simulink model "sensor_diagnosis"  (R2018b)
settings: Solver=FixedStepAuto  StartTime=0.0  StopTime=2000  FixedStep=0.02  RelTol=1e-3
values from neighbouring files (symbols this model uses):
  R = 0.003*eye(size(C,1))    [Com_of_kalman_gain.m]    (also in Copy_of_kalman_gain.m = diag(y_noise.^2); MM_HKF.m = diag(y_svar.^2); MM_based.m = diag(y_svar.^2); act_fault_of_kalman_gain.m = 0.02^2*eye(size(C,1)))
undefined symbols (not defined in the file or in its folder): piece
libraries: sharedschedule x121, dspsigattribs x22, commchan3 x1, dsparch4 x1, simulink x1
(part 1 of 2)
settings Model: Creator=mmm  LastModifiedBy=ma

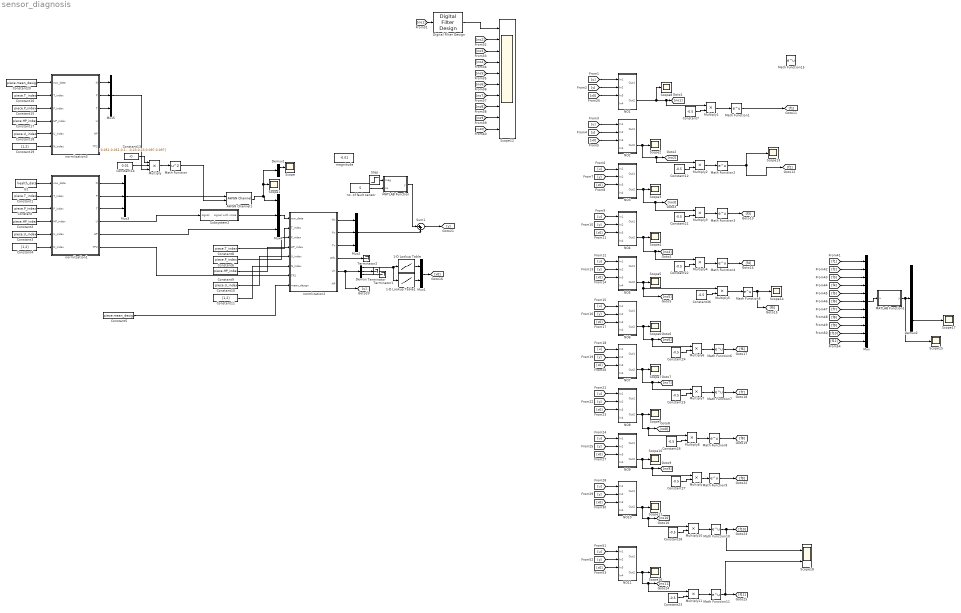
== system sensor_diagnosis ==
  1-D Lookup Table : Lookup_n-D  NumberOfTableDimensions=1  BreakpointsForDimension1=piece.Wf_stable_(:,1)  Table=piece.Nl  InterpMethod=Cubic spline  ExtrapMethod=Cubic spline  InternalRulePriority=Speed  RndMeth=Simplest  InputSameDT=on
  1-D Lookup Table1 : Lookup_n-D  NumberOfTableDimensions=1  BreakpointsForDimension1=piece.Wf_stable_(:,1)  Table=piece.N_stable_(:,2)  InterpMethod=Cubic spline  ExtrapMethod=Cubic spline  InternalRulePriority=Speed  RndMeth=Simplest  InputSameDT=on
  AWGN Channel1 : commchan3/AWGN Channel  InputProcessing=Columns as channels (frame based)  seed=11:20  noiseMode=Variance from port  EbNodB=10  EsNodB=10  SNRdB=10  bitsPerSym=1  Ps=1  Tsym=1  variance=[2.55,7.5,0.03,0.03,0.3,0.3,0.15,0.15,0.45,0.45].^2
  Constant : Constant  Value=piece.P_index  VectorParams1D=off
  Constant1 : Constant  Value=piece.T_index  VectorParams1D=off
  Constant10 : Constant  Value=piece.U_index  VectorParams1D=off
  Constant11 : Constant  Value=[1,2]  VectorParams1D=off
  Constant{7,12,21..28,36} (11 alike) : Constant  Value=-0.5
  Constant13 : Constant  Value=[0.051,0.051,0.164,0.164,0.15,0.15,0.23,0.23,0.097,0.097]
  Constant14 : Constant  Value=0.01
  Constant15 : Constant  Value=piece.P_index  VectorParams1D=off
  Constant16 : Constant  Value=piece.T_index  VectorParams1D=off
  Constant17 : Constant  Value=piece.HP_index  VectorParams1D=off
  Constant18 : Constant  Value=piece.U_index  VectorParams1D=off
  Constant19 : Constant  Value=[1,2]  VectorParams1D=off
  Constant2 : Constant  Value=piece.HP_index  VectorParams1D=off
  Constant20 : Constant  Value=piece.mean_design  VectorParams1D=off
  Constant3 : Constant  Value=piece.U_index  VectorParams1D=off
  Constant4 : Constant  Value=[1,2]  VectorParams1D=off
  Constant5 : Constant  Value=piece.mean_design  VectorParams1D=off
  Constant6 : Constant  Value=piece.P_index  VectorParams1D=off
  Constant8 : Constant  Value=piece.T_index  VectorParams1D=off
  Constant9 : Constant  Value=piece.HP_index  VectorParams1D=off
  Demux : Demux  Outputs=3
  Demux1 : Demux  Outputs=[1,9]
  Demux2 : Demux  Outputs=10
  Digital Filter Design : dsparch4/Digital Filter Design  mwdsp_browser_bugfix_var=off
  MATLAB Function : MATLAB Function  TreatAsAtomicUnit=on
  MATLAB Function1 : MATLAB Function  TreatAsAtomicUnit=on
  Math Function : Math  Operator=square  SaturateOnIntegerOverflow=on
  Math Function{1..11,15} (12 alike) : Math  SaturateOnIntegerOverflow=on
  Multiply : Product  Inputs=3
  Multiply{1..11} (11 alike) : Product
  Mux : Mux  Inputs=11
  Mux1 : Mux  Inputs=2
  Mux{2..5} (4 alike) : Mux  Inputs=3
  NO1 : Subsystem
  NO10 : Subsystem
  NO11 : Subsystem
  NO2 : Subsystem
  NO3 : Subsystem
  NO4 : Subsystem
  NO5 : Subsystem
  NO6 : Subsystem
  NO7 : Subsystem
  NO8 : Subsystem
  NO9 : Subsystem
  Scope{,1..11,13..17} (17 alike) : Scope
  Scope12 : Scope  NumInputPorts=10
  Scope18 : Scope  NumInputPorts=2
  Step : Step  Time=300  After=-0.02  SampleTime=0
  Subsystem2 : Subsystem
  Sum1 : Sum  Inputs=|++
  Terminator : Terminator
  Terminator1 : Terminator
  Terminator2 : Terminator
  U2 : FromWorkspace  VariableName=health_data  SampleTime=0.02  Interpolate=off  OutputAfterFinalValue=Holding final value
  magnitude : Constant  Value=-0.01
  no. of fault sensor : Constant  Value=5
  normlization1 : MATLAB Function  TreatAsAtomicUnit=on
  normlization2 : MATLAB Function  TreatAsAtomicUnit=on
  normlization3 : MATLAB Function  TreatAsAtomicUnit=on
  wires:
  Constant4/1 -> normlization1/6(N_index)
  Constant2/1 -> normlization1/4(HP_index)
  Constant3/1 -> normlization1/5(U_index)
  Constant1/1 -> normlization1/2(T_index)
  U2/1 -> normlization1/1(row_data)
  Constant/1 -> normlization1/3(P_index)
  Demux/1 -> 1-D Lookup Table1/1, 1-D Lookup Table/1
  Demux/2 -> Terminator/1
  Demux/3 -> Terminator1/1
  1-D Lookup Table/1 -> Mux1/1
  1-D Lookup Table1/1 -> Mux1/2
  Mux1/1 -> [x0]
  normlization2/5(Un) -> Demux/1, [u]
  Mux2/1 -> Sum1/2
  Sum1/1 -> [y]
  normlization1/1(N) -> Mux3/1
  normlization1/2(P) -> Mux3/2
  normlization1/3(T) -> Mux3/3
  Constant5/1 -> normlization2/8(mean_design)
  Mux3/1 -> AWGN Channel1/1
  normlization1/5(HP) -> Mux4/3
  Mux4/1 -> normlization2/1(row_data)
  Constant8/1 -> normlization2/2(T_index)
  Constant6/1 -> normlization2/3(P_index)
  Constant9/1 -> normlization2/4(HP_index)
  Constant10/1 -> normlization2/5(U_index)
  Constant11/1 -> normlization2/6(N_index)
  normlization2/1(Nn) -> Mux2/1
  normlization2/2(Pn) -> Mux2/2
  normlization2/3(Tn) -> Mux2/3
  normlization1/4(U) -> Subsystem2/1(signal)
  Subsystem2/1(signal with noise) -> Mux4/2
  normlization2/4(Wfn) -> Terminator2/1
  normlization1/6(TP2) -> normlization2/7(TP2)
  Demux1/1 -> Scope/1
  Constant13/1 -> Multiply/1
  Constant14/1 -> Multiply/2
  Multiply/1 -> Math Function/1
  Math Function/1 -> AWGN Channel1/2
  AWGN Channel1/1 -> Scope1/1, Demux1/1, Mux4/1
  Constant15/1 -> normlization3/3(P_index)
  Constant20/1 -> normlization3/1(row_data)
  Constant16/1 -> normlization3/2(T_index)
  Constant18/1 -> normlization3/5(U_index)
  Constant17/1 -> normlization3/4(HP_index)
  Constant19/1 -> normlization3/6(N_index)
  normlization3/1(N) -> Mux5/1
  normlization3/2(P) -> Mux5/2
  normlization3/3(T) -> Mux5/3
  Mux5/1 -> Multiply/3
  [u] -> NO1/1(In1)
  [y] -> NO1/2(In2)
  [x0] -> NO1/3(In3)
  NO1/2(Out2) -> Scope8/1, Multiply1/1, [no1]
  [u] -> NO2/1(In1)
  [y] -> NO2/2(In2)
  [x0] -> NO2/3(In3)
  [u] -> NO3/1(In1)
  [y] -> NO3/2(In2)
  [x0] -> NO3/3(In3)
  [x0] -> NO4/3(In3)
  [y] -> NO4/2(In2)
  [u] -> NO4/1(In1)
  [x0] -> NO5/3(In3)
  [y] -> NO5/2(In2)
  [u] -> NO5/1(In1)
  [x0] -> NO6/3(In3)
  [y] -> NO6/2(In2)
  [u] -> NO6/1(In1)
  [x0] -> NO7/3(In3)
  [y] -> NO7/2(In2)
  [u] -> NO7/1(In1)
  [x0] -> NO8/3(In3)
  [y] -> NO8/2(In2)
  [u] -> NO8/1(In1)
  [x0] -> NO9/3(In3)
  [y] -> NO9/2(In2)
  [u] -> NO9/1(In1)
  [x0] -> NO10/3(In3)
  [y] -> NO10/2(In2)
  [u] -> NO10/1(In1)
  [no2] -> Scope12/2
  [no3] -> Scope12/3
  [no4] -> Scope12/4
  [no5] -> Scope12/5
  [no6] -> Scope12/6
  [no7] -> Scope12/7
  [no8] -> Scope12/8
  [no9] -> Scope12/9
  [no10] -> Scope12/10
  no. of fault sensor/1 -> MATLAB Function/2(no)
  MATLAB Function/1(y) -> Sum1/1
  Step/1 -> MATLAB Function/1(mag)
  Constant7/1 -> Multiply1/2
  Multiply1/1 -> Math Function1/1
  Multiply2/1 -> Math Function2/1
  NO2/2(Out2) -> Multiply2/1, [no2], Scope2/1
  Constant12/1 -> Multiply2/2
  Multiply3/1 -> Math Function3/1
  NO3/2(Out2) -> Multiply3/1, [no3], Scope3/1
  Constant21/1 -> Multiply3/2
  Multiply4/1 -> Math Function4/1
  NO4/2(Out2) -> Multiply4/1, [no4], Scope4/1
  Constant22/1 -> Multiply4/2
  NO5/2(Out2) -> [no5], Multiply5/1, Scope5/1
  Multiply6/1 -> Math Function6/1
  NO6/2(Out2) -> Multiply6/1, [no6], Scope6/1
  Constant24/1 -> Multiply6/2
  Multiply7/1 -> Math Function7/1
  NO7/2(Out2) -> Multiply7/1, [no7], Scope7/1
  Constant25/1 -> Multiply7/2
  Multiply8/1 -> Math Function8/1
  NO8/2(Out2) -> Multiply8/1, [no8], Scope9/1
  Constant26/1 -> Multiply8/2
  Multiply9/1 -> Math Function9/1
  NO9/2(Out2) -> Multiply9/1, [no9], Scope10/1
  Constant27/1 -> Multiply9/2
  Multiply10/1 -> Math Function10/1
  NO10/2(Out2) -> Multiply10/1, [no10], Scope11/1
  Constant28/1 -> Multiply10/2
  Multiply5/1 -> Math Function5/1
  Constant36/1 -> Multiply5/2
  [no1] -> Digital Filter Design/1
  Digital Filter Design/1 -> Scope12/1
  Math Function1/1 -> [f1]
  Math Function5/1 -> [f5], Scope14/1
  Math Function2/1 -> [f2], Scope13/1
  Math Function3/1 -> [f3]
  Math Function4/1 -> [f4]
  Math Function6/1 -> [f6]
  Math Function7/1 -> [f7]
  Math Function8/1 -> [f8]
  Math Function9/1 -> [f9]
  Math Function10/1 -> Scope18/1, [f10]
  [f1] -> Mux/1
  [f2] -> Mux/2
  [f3] -> Mux/3
  [f4] -> Mux/4
  [f5] -> Mux/5
  [f6] -> Mux/6
  [f7] -> Mux/7
  [f8] -> Mux/8
  [f9] -> Mux/9
  [f10] -> Mux/10
  Mux/1 -> MATLAB Function1/1(u)
  MATLAB Function1/1(y) -> Scope15/1, Demux2/1
  Math Function11/1 -> Scope18/2, [f11]
  Constant23/1 -> Multiply11/2
  NO11/2(Out2) -> Scope16/1, [no11], Multiply11/1
  Multiply11/1 -> Math Function11/1
  [y] -> NO11/2(In2)
  [x0] -> NO11/3(In3)
  [u] -> NO11/1(In1)
  [f11] -> Mux/11
  Demux2/9 -> Scope17/1

== system sensor_diagnosis/NO1 ==
  In1 : Inport
  In2 : Inport  Port=2
  In3 : Inport  Port=3
  In4 : Inport  Port=4
  A : sharedschedule/Interpolate Matrix(x)   matrix=piece.A  aMode=aMode
      settings: SourceProductName=Aerospace Blockset  SourceProductBaseCode=AE
  B : sharedschedule/Interpolate Matrix(x)   matrix=piece.B  aMode=aMode
      settings: SourceProductName=Aerospace Blockset  SourceProductBaseCode=AE
  C : sharedschedule/Interpolate Matrix(x)   matrix=piece.C  aMode=aMode
      settings: SourceProductName=Aerospace Blockset  SourceProductBaseCode=AE
  D : sharedschedule/Interpolate Matrix(x)   matrix=piece.D  aMode=aMode
      settings: SourceProductName=Aerospace Blockset  SourceProductBaseCode=AE
  K1 : sharedschedule/Interpolate Matrix(x)   matrix=piece.K_s  aMode=aMode
      settings: SourceProductName=Aerospace Blockset  SourceProductBaseCode=AE
  K2 : sharedschedule/Interpolate Matrix(x)   matrix=piece.S_s  aMode=aMode
      settings: SourceProductName=Aerospace Blockset  SourceProductBaseCode=AE
  L : sharedschedule/Interpolate Matrix(x)   matrix=piece.L  aMode=aMode
      settings: SourceProductName=Aerospace Blockset  SourceProductBaseCode=AE
  M : sharedschedule/Interpolate Matrix(x)   matrix=piece.M  aMode=aMode
      settings: SourceProductName=Aerospace Blockset  SourceProductBaseCode=AE
  Matrix Divide1 : Product  Inputs=*/  Multiplication=Matrix(*)
  MatrixMultiply1 : Product  Multiplication=Matrix(*)
  Minus1 : Sum  Inputs=+-
  Minus5 : Sum  Inputs=+-
  Prelookup : PreLookup  BreakpointsData=piece.Nl  BreakpointObject=Nl  ExtrapMethod=Linear  UseLastBreakpoint=on  DiagnosticForOutOfRangeInput=Warning
  Scope2 : Scope
  Selector : Selector  InputPortWidth=2  IndexOptions=Index vector (dialog)  Indices=[1]  OutputSizes=1
  Transpose3 : Math  Operator=transpose  SaturateOnIntegerOverflow=on
  kalman filter1 : Subsystem
  steadyOutput : sharedschedule/Interpolate Matrix(x)   matrix=piece.steadyOutput  aMode=aMode
      settings: SourceProductName=Aerospace Blockset  SourceProductBaseCode=AE
  steadyState : sharedschedule/Interpolate Matrix(x)   matrix=piece.steadyState  aMode=aMode
      settings: SourceProductName=Aerospace Blockset  SourceProductBaseCode=AE
  steadyinput : sharedschedule/Interpolate Matrix(x)   matrix=piece.steadyInput  aMode=aMode
      settings: SourceProductName=Aerospace Blockset  SourceProductBaseCode=AE
  Out1 : Outport
  Out2 : Outport  Port=2
  wires:
  D/1 -> kalman filter1/4(D)
  Prelookup/1 -> K2/1, K1/1, M/1, L/1, steadyState/1, steadyinput/1, steadyOutput/1, D/1, C/1, B/1, A/1
  In4/1 -> kalman filter1/12(P)
  kalman filter1/3(Y_error) -> Transpose3/1, MatrixMultiply1/2, Scope2/1
  B/1 -> kalman filter1/2(B)
  Prelookup/2 -> A/2, steadyState/2, K2/2, K1/2, M/2, L/2, steadyinput/2, steadyOutput/2, D/2, C/2, B/2
  Selector/1 -> Prelookup/1
  steadyState/1 -> kalman filter1/9(Xtrim)
  Transpose3/1 -> Matrix Divide1/1
  Matrix Divide1/1 -> MatrixMultiply1/1
  L/1 -> kalman filter1/10(L)
  C/1 -> kalman filter1/3(C)
  Minus5/1 -> kalman filter1/7(Y)
  kalman filter1/2(Y_es) -> Out1/1
  Minus1/1 -> kalman filter1/8(U)
  kalman filter1/1(X_es) -> Selector/1
  steadyinput/1 -> Minus1/2
  K1/1 -> kalman filter1/5(K)
  steadyOutput/1 -> Minus5/2
  A/1 -> kalman filter1/1(A)
  MatrixMultiply1/1 -> Out2/1
  M/1 -> kalman filter1/11(M)
  In3/1 -> kalman filter1/6(x0)
  In2/1 -> Minus5/1
  In1/1 -> Minus1/1
  K2/1 -> Matrix Divide1/2

== system sensor_diagnosis/NO10 ==
  In1 : Inport
  In2 : Inport  Port=2
  In3 : Inport  Port=3
  In4 : Inport  Port=4
  A : sharedschedule/Interpolate Matrix(x)   matrix=piece.A  aMode=aMode
      settings: SourceProductName=Aerospace Blockset  SourceProductBaseCode=AE
  B : sharedschedule/Interpolate Matrix(x)   matrix=piece.B  aMode=aMode
      settings: SourceProductName=Aerospace Blockset  SourceProductBaseCode=AE
  C : sharedschedule/Interpolate Matrix(x)   matrix=piece.C  aMode=aMode
      settings: SourceProductName=Aerospace Blockset  SourceProductBaseCode=AE
  Constant7 : Constant  Value=R  VectorParams1D=off
  D : sharedschedule/Interpolate Matrix(x)   matrix=piece.D  aMode=aMode
      settings: SourceProductName=Aerospace Blockset  SourceProductBaseCode=AE
  K1 : sharedschedule/Interpolate Matrix(x)   matrix=piece.K_s  aMode=aMode
      settings: SourceProductName=Aerospace Blockset  SourceProductBaseCode=AE
  K2 : sharedschedule/Interpolate Matrix(x)   matrix=piece.S_s  aMode=aMode
      settings: SourceProductName=Aerospace Blockset  SourceProductBaseCode=AE
  L : sharedschedule/Interpolate Matrix(x)   matrix=piece.L  aMode=aMode
      settings: SourceProductName=Aerospace Blockset  SourceProductBaseCode=AE
  M : sharedschedule/Interpolate Matrix(x)   matrix=piece.M  aMode=aMode
      settings: SourceProductName=Aerospace Blockset  SourceProductBaseCode=AE
  Matrix Divide1 : Product  Inputs=*/  Multiplication=Matrix(*)
  MatrixMultiply1 : Product  Multiplication=Matrix(*)
  Minus1 : Sum  Inputs=+-
  Minus5 : Sum  Inputs=+-
  Prelookup : PreLookup  BreakpointsData=piece.Nl  BreakpointObject=Nl  ExtrapMethod=Linear  UseLastBreakpoint=on  DiagnosticForOutOfRangeInput=Warning
  Scope2 : Scope
  Selector : Selector  InputPortWidth=2  IndexOptions=Index vector (dialog)  Indices=[1]  OutputSizes=1
  Transpose3 : Math  Operator=transpose  SaturateOnIntegerOverflow=on
  kalman filter1 : Subsystem
  steadyOutput : sharedschedule/Interpolate Matrix(x)   matrix=piece.steadyOutput  aMode=aMode
      settings: SourceProductName=Aerospace Blockset  SourceProductBaseCode=AE
  steadyState : sharedschedule/Interpolate Matrix(x)   matrix=piece.steadyState  aMode=aMode
      settings: SourceProductName=Aerospace Blockset  SourceProductBaseCode=AE
  steadyinput : sharedschedule/Interpolate Matrix(x)   matrix=piece.steadyInput  aMode=aMode
      settings: SourceProductName=Aerospace Blockset  SourceProductBaseCode=AE
  Out1 : Outport
  Out2 : Outport  Port=2
  wires:
  D/1 -> kalman filter1/4(D)
  In4/1 -> kalman filter1/12(P)
  kalman filter1/3(Y_error) -> Transpose3/1, MatrixMultiply1/2, Scope2/1
  B/1 -> kalman filter1/2(B)
  Prelookup/2 -> A/2, steadyState/2, K2/2, K1/2, M/2, L/2, steadyinput/2, steadyOutput/2, D/2, C/2, B/2
  Selector/1 -> Prelookup/1
  steadyState/1 -> kalman filter1/9(Xtrim)
  Transpose3/1 -> Matrix Divide1/1
  Matrix Divide1/1 -> MatrixMultiply1/1
  L/1 -> kalman filter1/10(L)
  C/1 -> kalman filter1/3(C)
  Minus5/1 -> kalman filter1/7(Y)
  kalman filter1/2(Y_es) -> Out1/1
  Minus1/1 -> kalman filter1/8(U)
  kalman filter1/1(X_es) -> Selector/1
  steadyinput/1 -> Minus1/2
  K1/1 -> kalman filter1/5(K)
  steadyOutput/1 -> Minus5/2
  A/1 -> kalman filter1/1(A)
  MatrixMultiply1/1 -> Out2/1
  M/1 -> kalman filter1/11(M)
  In3/1 -> kalman filter1/6(x0)
  In2/1 -> Minus5/1
  In1/1 -> Minus1/1
  Prelookup/1 -> K2/1, K1/1, M/1, L/1, steadyState/1, steadyinput/1, steadyOutput/1, D/1, C/1, B/1, A/1
  K2/1 -> Matrix Divide1/2

== system sensor_diagnosis/NO11 ==
  In1 : Inport
  In2 : Inport  Port=2
  In3 : Inport  Port=3
  In4 : Inport  Port=4
  A : sharedschedule/Interpolate Matrix(x)   matrix=piece.A  aMode=aMode
      settings: SourceProductName=Aerospace Blockset  SourceProductBaseCode=AE
  B : sharedschedule/Interpolate Matrix(x)   matrix=piece.B  aMode=aMode
      settings: SourceProductName=Aerospace Blockset  SourceProductBaseCode=AE
  C : sharedschedule/Interpolate Matrix(x)   matrix=piece.C  aMode=aMode
      settings: SourceProductName=Aerospace Blockset  SourceProductBaseCode=AE
  Constant7 : Constant  Value=R  VectorParams1D=off
  D : sharedschedule/Interpolate Matrix(x)   matrix=piece.D  aMode=aMode
      settings: SourceProductName=Aerospace Blockset  SourceProductBaseCode=AE
  K1 : sharedschedule/Interpolate Matrix(x)   matrix=piece.K_s  aMode=aMode
      settings: SourceProductName=Aerospace Blockset  SourceProductBaseCode=AE
  K2 : sharedschedule/Interpolate Matrix(x)   matrix=piece.S_s  aMode=aMode
      settings: SourceProductName=Aerospace Blockset  SourceProductBaseCode=AE
  L : sharedschedule/Interpolate Matrix(x)   matrix=piece.L  aMode=aMode
      settings: SourceProductName=Aerospace Blockset  SourceProductBaseCode=AE
  M : sharedschedule/Interpolate Matrix(x)   matrix=piece.M  aMode=aMode
      settings: SourceProductName=Aerospace Blockset  SourceProductBaseCode=AE
  Matrix Divide1 : Product  Inputs=*/  Multiplication=Matrix(*)
  MatrixMultiply1 : Product  Multiplication=Matrix(*)
  Minus1 : Sum  Inputs=+-
  Minus5 : Sum  Inputs=+-
  Prelookup : PreLookup  BreakpointsData=piece.Nl  BreakpointObject=Nl  ExtrapMethod=Linear  UseLastBreakpoint=on  DiagnosticForOutOfRangeInput=Warning
  Scope2 : Scope
  Selector : Selector  InputPortWidth=2  IndexOptions=Index vector (dialog)  Indices=[1]  OutputSizes=1
  Transpose3 : Math  Operator=transpose  SaturateOnIntegerOverflow=on
  kalman filter1 : Subsystem
  steadyOutput : sharedschedule/Interpolate Matrix(x)   matrix=piece.steadyOutput  aMode=aMode
      settings: SourceProductName=Aerospace Blockset  SourceProductBaseCode=AE
  steadyState : sharedschedule/Interpolate Matrix(x)   matrix=piece.steadyState  aMode=aMode
      settings: SourceProductName=Aerospace Blockset  SourceProductBaseCode=AE
  steadyinput : sharedschedule/Interpolate Matrix(x)   matrix=piece.steadyInput  aMode=aMode
      settings: SourceProductName=Aerospace Blockset  SourceProductBaseCode=AE
  Out1 : Outport
  Out2 : Outport  Port=2
  wires:
  K2/1 -> Matrix Divide1/2
  Prelookup/1 -> A/1, B/1, C/1, D/1, steadyOutput/1, steadyinput/1, steadyState/1, L/1, M/1, K1/1, K2/1
  In1/1 -> Minus1/1
  In2/1 -> Minus5/1
  In3/1 -> kalman filter1/6(x0)
  M/1 -> kalman filter1/11(M)
  MatrixMultiply1/1 -> Out2/1
  A/1 -> kalman filter1/1(A)
  steadyOutput/1 -> Minus5/2
  K1/1 -> kalman filter1/5(K)
  steadyinput/1 -> Minus1/2
  kalman filter1/1(X_es) -> Selector/1
  Minus1/1 -> kalman filter1/8(U)
  kalman filter1/2(Y_es) -> Out1/1
  Minus5/1 -> kalman filter1/7(Y)
  C/1 -> kalman filter1/3(C)
  L/1 -> kalman filter1/10(L)
  Matrix Divide1/1 -> MatrixMultiply1/1
  Transpose3/1 -> Matrix Divide1/1
  steadyState/1 -> kalman filter1/9(Xtrim)
  Selector/1 -> Prelookup/1
  Prelookup/2 -> B/2, C/2, D/2, steadyOutput/2, steadyinput/2, L/2, M/2, K1/2, K2/2, steadyState/2, A/2
  B/1 -> kalman filter1/2(B)
  kalman filter1/3(Y_error) -> Scope2/1, MatrixMultiply1/2, Transpose3/1
  In4/1 -> kalman filter1/12(P)
  D/1 -> kalman filter1/4(D)

== system sensor_diagnosis/NO2 ==
  In1 : Inport
  In2 : Inport  Port=2
  In3 : Inport  Port=3
  In4 : Inport  Port=4
  A : sharedschedule/Interpolate Matrix(x)   matrix=piece.A  aMode=aMode
      settings: SourceProductName=Aerospace Blockset  SourceProductBaseCode=AE
  B : sharedschedule/Interpolate Matrix(x)   matrix=piece.B  aMode=aMode
      settings: SourceProductName=Aerospace Blockset  SourceProductBaseCode=AE
  C : sharedschedule/Interpolate Matrix(x)   matrix=piece.C  aMode=aMode
      settings: SourceProductName=Aerospace Blockset  SourceProductBaseCode=AE
  D : sharedschedule/Interpolate Matrix(x)   matrix=piece.D  aMode=aMode
      settings: SourceProductName=Aerospace Blockset  SourceProductBaseCode=AE
  K1 : sharedschedule/Interpolate Matrix(x)   matrix=piece.K_s  aMode=aMode
      settings: SourceProductName=Aerospace Blockset  SourceProductBaseCode=AE
  K2 : sharedschedule/Interpolate Matrix(x)   matrix=piece.S_s  aMode=aMode
      settings: SourceProductName=Aerospace Blockset  SourceProductBaseCode=AE
  L : sharedschedule/Interpolate Matrix(x)   matrix=piece.L  aMode=aMode
      settings: SourceProductName=Aerospace Blockset  SourceProductBaseCode=AE
  M : sharedschedule/Interpolate Matrix(x)   matrix=piece.M  aMode=aMode
      settings: SourceProductName=Aerospace Blockset  SourceProductBaseCode=AE
  Matrix Divide1 : Product  Inputs=*/  Multiplication=Matrix(*)
  MatrixMultiply1 : Product  Multiplication=Matrix(*)
  Minus1 : Sum  Inputs=+-
  Minus5 : Sum  Inputs=+-
  Prelookup : PreLookup  BreakpointsData=piece.Nl  BreakpointObject=Nl  ExtrapMethod=Linear  UseLastBreakpoint=on  DiagnosticForOutOfRangeInput=Warning
  Scope2 : Scope
  Selector : Selector  InputPortWidth=2  IndexOptions=Index vector (dialog)  Indices=[1]  OutputSizes=1
  Transpose3 : Math  Operator=transpose  SaturateOnIntegerOverflow=on
  kalman filter1 : Subsystem
  steadyOutput : sharedschedule/Interpolate Matrix(x)   matrix=piece.steadyOutput  aMode=aMode
      settings: SourceProductName=Aerospace Blockset  SourceProductBaseCode=AE
  steadyState : sharedschedule/Interpolate Matrix(x)   matrix=piece.steadyState  aMode=aMode
      settings: SourceProductName=Aerospace Blockset  SourceProductBaseCode=AE
  steadyinput : sharedschedule/Interpolate Matrix(x)   matrix=piece.steadyInput  aMode=aMode
      settings: SourceProductName=Aerospace Blockset  SourceProductBaseCode=AE
  Out1 : Outport
  Out2 : Outport  Port=2
  wires:
  D/1 -> kalman filter1/4(D)
  Prelookup/1 -> K2/1, K1/1, M/1, L/1, steadyState/1, steadyinput/1, steadyOutput/1, D/1, C/1, B/1, A/1
  In4/1 -> kalman filter1/12(P)
  kalman filter1/3(Y_error) -> Transpose3/1, MatrixMultiply1/2, Scope2/1
  B/1 -> kalman filter1/2(B)
  Prelookup/2 -> A/2, steadyState/2, K2/2, K1/2, M/2, L/2, steadyinput/2, steadyOutput/2, D/2, C/2, B/2
  Selector/1 -> Prelookup/1
  steadyState/1 -> kalman filter1/9(Xtrim)
  Transpose3/1 -> Matrix Divide1/1
  Matrix Divide1/1 -> MatrixMultiply1/1
  L/1 -> kalman filter1/10(L)
  C/1 -> kalman filter1/3(C)
  Minus5/1 -> kalman filter1/7(Y)
  kalman filter1/2(Y_es) -> Out1/1
  Minus1/1 -> kalman filter1/8(U)
  K2/1 -> Matrix Divide1/2
  kalman filter1/1(X_es) -> Selector/1
  steadyinput/1 -> Minus1/2
  K1/1 -> kalman filter1/5(K)
  steadyOutput/1 -> Minus5/2
  A/1 -> kalman filter1/1(A)
  MatrixMultiply1/1 -> Out2/1
  M/1 -> kalman filter1/11(M)
  In3/1 -> kalman filter1/6(x0)
  In2/1 -> Minus5/1
  In1/1 -> Minus1/1

== system sensor_diagnosis/NO3 ==
  In1 : Inport
  In2 : Inport  Port=2
  In3 : Inport  Port=3
  In4 : Inport  Port=4
  A : sharedschedule/Interpolate Matrix(x)   matrix=piece.A  aMode=aMode
      settings: SourceProductName=Aerospace Blockset  SourceProductBaseCode=AE
  B : sharedschedule/Interpolate Matrix(x)   matrix=piece.B  aMode=aMode
      settings: SourceProductName=Aerospace Blockset  SourceProductBaseCode=AE
  C : sharedschedule/Interpolate Matrix(x)   matrix=piece.C  aMode=aMode
      settings: SourceProductName=Aerospace Blockset  SourceProductBaseCode=AE
  Constant7 : Constant  Value=R  VectorParams1D=off
  D : sharedschedule/Interpolate Matrix(x)   matrix=piece.D  aMode=aMode
      settings: SourceProductName=Aerospace Blockset  SourceProductBaseCode=AE
  K1 : sharedschedule/Interpolate Matrix(x)   matrix=piece.K_s  aMode=aMode
      settings: SourceProductName=Aerospace Blockset  SourceProductBaseCode=AE
  K2 : sharedschedule/Interpolate Matrix(x)   matrix=piece.S_s  aMode=aMode
      settings: SourceProductName=Aerospace Blockset  SourceProductBaseCode=AE
  L : sharedschedule/Interpolate Matrix(x)   matrix=piece.L  aMode=aMode
      settings: SourceProductName=Aerospace Blockset  SourceProductBaseCode=AE
  M : sharedschedule/Interpolate Matrix(x)   matrix=piece.M  aMode=aMode
      settings: SourceProductName=Aerospace Blockset  SourceProductBaseCode=AE
  Matrix Divide1 : Product  Inputs=*/  Multiplication=Matrix(*)
  MatrixMultiply1 : Product  Multiplication=Matrix(*)
  Minus1 : Sum  Inputs=+-
  Minus5 : Sum  Inputs=+-
  Prelookup : PreLookup  BreakpointsData=piece.Nl  BreakpointObject=Nl  ExtrapMethod=Linear  UseLastBreakpoint=on  DiagnosticForOutOfRangeInput=Warning
  Scope2 : Scope
  Selector : Selector  InputPortWidth=2  IndexOptions=Index vector (dialog)  Indices=[1]  OutputSizes=1
  Transpose3 : Math  Operator=transpose  SaturateOnIntegerOverflow=on
  kalman filter1 : Subsystem
  steadyOutput : sharedschedule/Interpolate Matrix(x)   matrix=piece.steadyOutput  aMode=aMode
      settings: SourceProductName=Aerospace Blockset  SourceProductBaseCode=AE
  steadyState : sharedschedule/Interpolate Matrix(x)   matrix=piece.steadyState  aMode=aMode
      settings: SourceProductName=Aerospace Blockset  SourceProductBaseCode=AE
  steadyinput : sharedschedule/Interpolate Matrix(x)   matrix=piece.steadyInput  aMode=aMode
      settings: SourceProductName=Aerospace Blockset  SourceProductBaseCode=AE
  Out1 : Outport
  Out2 : Outport  Port=2
  wires:
  D/1 -> kalman filter1/4(D)
  Prelookup/1 -> K2/1, K1/1, M/1, L/1, steadyState/1, steadyinput/1, steadyOutput/1, D/1, C/1, B/1, A/1
  In4/1 -> kalman filter1/12(P)
  kalman filter1/3(Y_error) -> Transpose3/1, MatrixMultiply1/2, Scope2/1
  B/1 -> kalman filter1/2(B)
  Prelookup/2 -> A/2, steadyState/2, K2/2, K1/2, M/2, L/2, steadyinput/2, steadyOutput/2, D/2, C/2, B/2
  Selector/1 -> Prelookup/1
  steadyState/1 -> kalman filter1/9(Xtrim)
  Transpose3/1 -> Matrix Divide1/1
  Matrix Divide1/1 -> MatrixMultiply1/1
  L/1 -> kalman filter1/10(L)
  C/1 -> kalman filter1/3(C)
  Minus5/1 -> kalman filter1/7(Y)
  kalman filter1/2(Y_es) -> Out1/1
  Minus1/1 -> kalman filter1/8(U)
  kalman filter1/1(X_es) -> Selector/1
  steadyinput/1 -> Minus1/2
  K1/1 -> kalman filter1/5(K)
  steadyOutput/1 -> Minus5/2
  A/1 -> kalman filter1/1(A)
  MatrixMultiply1/1 -> Out2/1
  M/1 -> kalman filter1/11(M)
  In3/1 -> kalman filter1/6(x0)
  In2/1 -> Minus5/1
  In1/1 -> Minus1/1
  K2/1 -> Matrix Divide1/2

== system sensor_diagnosis/NO4 ==
  In1 : Inport
  In2 : Inport  Port=2
  In3 : Inport  Port=3
  In4 : Inport  Port=4
  A : sharedschedule/Interpolate Matrix(x)   matrix=piece.A  aMode=aMode
      settings: SourceProductName=Aerospace Blockset  SourceProductBaseCode=AE
  B : sharedschedule/Interpolate Matrix(x)   matrix=piece.B  aMode=aMode
      settings: SourceProductName=Aerospace Blockset  SourceProductBaseCode=AE
  C : sharedschedule/Interpolate Matrix(x)   matrix=piece.C  aMode=aMode
      settings: SourceProductName=Aerospace Blockset  SourceProductBaseCode=AE
  Constant7 : Constant  Value=R  VectorParams1D=off
  D : sharedschedule/Interpolate Matrix(x)   matrix=piece.D  aMode=aMode
      settings: SourceProductName=Aerospace Blockset  SourceProductBaseCode=AE
  K1 : sharedschedule/Interpolate Matrix(x)   matrix=piece.K_s  aMode=aMode
      settings: SourceProductName=Aerospace Blockset  SourceProductBaseCode=AE
  K2 : sharedschedule/Interpolate Matrix(x)   matrix=piece.S_s  aMode=aMode
      settings: SourceProductName=Aerospace Blockset  SourceProductBaseCode=AE
  L : sharedschedule/Interpolate Matrix(x)   matrix=piece.L  aMode=aMode
      settings: SourceProductName=Aerospace Blockset  SourceProductBaseCode=AE
  M : sharedschedule/Interpolate Matrix(x)   matrix=piece.M  aMode=aMode
      settings: SourceProductName=Aerospace Blockset  SourceProductBaseCode=AE
  Matrix Divide1 : Product  Inputs=*/  Multiplication=Matrix(*)
  MatrixMultiply1 : Product  Multiplication=Matrix(*)
  Minus1 : Sum  Inputs=+-
  Minus5 : Sum  Inputs=+-
  Prelookup : PreLookup  BreakpointsData=piece.Nl  BreakpointObject=Nl  ExtrapMethod=Linear  UseLastBreakpoint=on  DiagnosticForOutOfRangeInput=Warning
  Scope2 : Scope
  Selector : Selector  InputPortWidth=2  IndexOptions=Index vector (dialog)  Indices=[1]  OutputSizes=1
  Transpose3 : Math  Operator=transpose  SaturateOnIntegerOverflow=on
  kalman filter1 : Subsystem
  steadyOutput : sharedschedule/Interpolate Matrix(x)   matrix=piece.steadyOutput  aMode=aMode
      settings: SourceProductName=Aerospace Blockset  SourceProductBaseCode=AE
  steadyState : sharedschedule/Interpolate Matrix(x)   matrix=piece.steadyState  aMode=aMode
      settings: SourceProductName=Aerospace Blockset  SourceProductBaseCode=AE
  steadyinput : sharedschedule/Interpolate Matrix(x)   matrix=piece.steadyInput  aMode=aMode
      settings: SourceProductName=Aerospace Blockset  SourceProductBaseCode=AE
  Out1 : Outport
  Out2 : Outport  Port=2
  wires:
  D/1 -> kalman filter1/4(D)
  Prelookup/1 -> K2/1, K1/1, M/1, L/1, steadyState/1, steadyinput/1, steadyOutput/1, D/1, C/1, B/1, A/1
  In4/1 -> kalman filter1/12(P)
  kalman filter1/3(Y_error) -> Transpose3/1, MatrixMultiply1/2, Scope2/1
  B/1 -> kalman filter1/2(B)
  Prelookup/2 -> A/2, steadyState/2, K2/2, K1/2, M/2, L/2, steadyinput/2, steadyOutput/2, D/2, C/2, B/2
  Selector/1 -> Prelookup/1
  steadyState/1 -> kalman filter1/9(Xtrim)
  Transpose3/1 -> Matrix Divide1/1
  Matrix Divide1/1 -> MatrixMultiply1/1
  L/1 -> kalman filter1/10(L)
  C/1 -> kalman filter1/3(C)
  Minus5/1 -> kalman filter1/7(Y)
  kalman filter1/2(Y_es) -> Out1/1
  Minus1/1 -> kalman filter1/8(U)
  kalman filter1/1(X_es) -> Selector/1
  steadyinput/1 -> Minus1/2
  K1/1 -> kalman filter1/5(K)
  steadyOutput/1 -> Minus5/2
  A/1 -> kalman filter1/1(A)
  MatrixMultiply1/1 -> Out2/1
  M/1 -> kalman filter1/11(M)
  In3/1 -> kalman filter1/6(x0)
  In2/1 -> Minus5/1
  In1/1 -> Minus1/1
  K2/1 -> Matrix Divide1/2

== system sensor_diagnosis/NO5 ==
  In1 : Inport
  In2 : Inport  Port=2
  In3 : Inport  Port=3
  In4 : Inport  Port=4
  A : sharedschedule/Interpolate Matrix(x)   matrix=piece.A  aMode=aMode
      settings: SourceProductName=Aerospace Blockset  SourceProductBaseCode=AE
  B : sharedschedule/Interpolate Matrix(x)   matrix=piece.B  aMode=aMode
      settings: SourceProductName=Aerospace Blockset  SourceProductBaseCode=AE
  C : sharedschedule/Interpolate Matrix(x)   matrix=piece.C  aMode=aMode
      settings: SourceProductName=Aerospace Blockset  SourceProductBaseCode=AE
  Constant7 : Constant  Value=R  VectorParams1D=off
  D : sharedschedule/Interpolate Matrix(x)   matrix=piece.D  aMode=aMode
      settings: SourceProductName=Aerospace Blockset  SourceProductBaseCode=AE
  K1 : sharedschedule/Interpolate Matrix(x)   matrix=piece.K_s  aMode=aMode
      settings: SourceProductName=Aerospace Blockset  SourceProductBaseCode=AE
  K2 : sharedschedule/Interpolate Matrix(x)   matrix=piece.S_s  aMode=aMode
      settings: SourceProductName=Aerospace Blockset  SourceProductBaseCode=AE
  L : sharedschedule/Interpolate Matrix(x)   matrix=piece.L  aMode=aMode
      settings: SourceProductName=Aerospace Blockset  SourceProductBaseCode=AE
  M : sharedschedule/Interpolate Matrix(x)   matrix=piece.M  aMode=aMode
      settings: SourceProductName=Aerospace Blockset  SourceProductBaseCode=AE
  Matrix Divide1 : Product  Inputs=*/  Multiplication=Matrix(*)
  MatrixMultiply1 : Product  Multiplication=Matrix(*)
  Minus1 : Sum  Inputs=+-
  Minus5 : Sum  Inputs=+-
  Prelookup : PreLookup  BreakpointsData=piece.Nl  BreakpointObject=Nl  ExtrapMethod=Linear  UseLastBreakpoint=on  DiagnosticForOutOfRangeInput=Warning
  Scope2 : Scope
  Selector : Selector  InputPortWidth=2  IndexOptions=Index vector (dialog)  Indices=[1]  OutputSizes=1
  Transpose3 : Math  Operator=transpose  SaturateOnIntegerOverflow=on
  kalman filter1 : Subsystem
  steadyOutput : sharedschedule/Interpolate Matrix(x)   matrix=piece.steadyOutput  aMode=aMode
      settings: SourceProductName=Aerospace Blockset  SourceProductBaseCode=AE
  steadyState : sharedschedule/Interpolate Matrix(x)   matrix=piece.steadyState  aMode=aMode
      settings: SourceProductName=Aerospace Blockset  SourceProductBaseCode=AE
  steadyinput : sharedschedule/Interpolate Matrix(x)   matrix=piece.steadyInput  aMode=aMode
      settings: SourceProductName=Aerospace Blockset  SourceProductBaseCode=AE
  Out1 : Outport
  Out2 : Outport  Port=2
  wires:
  D/1 -> kalman filter1/4(D)
  Prelookup/1 -> K2/1, K1/1, M/1, L/1, steadyState/1, steadyinput/1, steadyOutput/1, D/1, C/1, B/1, A/1
  In4/1 -> kalman filter1/12(P)
  kalman filter1/3(Y_error) -> Transpose3/1, MatrixMultiply1/2, Scope2/1
  B/1 -> kalman filter1/2(B)
  Prelookup/2 -> A/2, steadyState/2, K2/2, K1/2, M/2, L/2, steadyinput/2, steadyOutput/2, D/2, C/2, B/2
  Selector/1 -> Prelookup/1
  steadyState/1 -> kalman filter1/9(Xtrim)
  Transpose3/1 -> Matrix Divide1/1
  Matrix Divide1/1 -> MatrixMultiply1/1
  L/1 -> kalman filter1/10(L)
  C/1 -> kalman filter1/3(C)
  Minus5/1 -> kalman filter1/7(Y)
  kalman filter1/2(Y_es) -> Out1/1
  Minus1/1 -> kalman filter1/8(U)
  kalman filter1/1(X_es) -> Selector/1
  steadyinput/1 -> Minus1/2
  K1/1 -> kalman filter1/5(K)
  steadyOutput/1 -> Minus5/2
  A/1 -> kalman filter1/1(A)
  MatrixMultiply1/1 -> Out2/1
  M/1 -> kalman filter1/11(M)
  In3/1 -> kalman filter1/6(x0)
  In2/1 -> Minus5/1
  In1/1 -> Minus1/1
  K2/1 -> Matrix Divide1/2

== system sensor_diagnosis/NO6 ==
  In1 : Inport
  In2 : Inport  Port=2
  In3 : Inport  Port=3
  In4 : Inport  Port=4
  A : sharedschedule/Interpolate Matrix(x)   matrix=piece.A  aMode=aMode
      settings: SourceProductName=Aerospace Blockset  SourceProductBaseCode=AE
  B : sharedschedule/Interpolate Matrix(x)   matrix=piece.B  aMode=aMode
      settings: SourceProductName=Aerospace Blockset  SourceProductBaseCode=AE
  C : sharedschedule/Interpolate Matrix(x)   matrix=piece.C  aMode=aMode
      settings: SourceProductName=Aerospace Blockset  SourceProductBaseCode=AE
  Constant7 : Constant  Value=R  VectorParams1D=off
  D : sharedschedule/Interpolate Matrix(x)   matrix=piece.D  aMode=aMode
      settings: SourceProductName=Aerospace Blockset  SourceProductBaseCode=AE
  K1 : sharedschedule/Interpolate Matrix(x)   matrix=piece.K_s  aMode=aMode
      settings: SourceProductName=Aerospace Blockset  SourceProductBaseCode=AE
  K2 : sharedschedule/Interpolate Matrix(x)   matrix=piece.S_s  aMode=aMode
      settings: SourceProductName=Aerospace Blockset  SourceProductBaseCode=AE
  L : sharedschedule/Interpolate Matrix(x)   matrix=piece.L  aMode=aMode
      settings: SourceProductName=Aerospace Blockset  SourceProductBaseCode=AE
  M : sharedschedule/Interpolate Matrix(x)   matrix=piece.M  aMode=aMode
      settings: SourceProductName=Aerospace Blockset  SourceProductBaseCode=AE
  Matrix Divide1 : Product  Inputs=*/  Multiplication=Matrix(*)
  MatrixMultiply1 : Product  Multiplication=Matrix(*)
  Minus1 : Sum  Inputs=+-
  Minus5 : Sum  Inputs=+-
  Prelookup : PreLookup  BreakpointsData=piece.Nl  BreakpointObject=Nl  ExtrapMethod=Linear  UseLastBreakpoint=on  DiagnosticForOutOfRangeInput=Warning
  Scope2 : Scope
  Selector : Selector  InputPortWidth=2  IndexOptions=Index vector (dialog)  Indices=[1]  OutputSizes=1
  Transpose3 : Math  Operator=transpose  SaturateOnIntegerOverflow=on
  kalman filter1 : Subsystem
  steadyOutput : sharedschedule/Interpolate Matrix(x)   matrix=piece.steadyOutput  aMode=aMode
      settings: SourceProductName=Aerospace Blockset  SourceProductBaseCode=AE
  steadyState : sharedschedule/Interpolate Matrix(x)   matrix=piece.steadyState  aMode=aMode
      settings: SourceProductName=Aerospace Blockset  SourceProductBaseCode=AE
  steadyinput : sharedschedule/Interpolate Matrix(x)   matrix=piece.steadyInput  aMode=aMode
      settings: SourceProductName=Aerospace Blockset  SourceProductBaseCode=AE
  Out1 : Outport
  Out2 : Outport  Port=2
  wires:
  D/1 -> kalman filter1/4(D)
  Prelookup/1 -> K2/1, K1/1, M/1, L/1, steadyState/1, steadyinput/1, steadyOutput/1, D/1, C/1, B/1, A/1
  In4/1 -> kalman filter1/12(P)
  kalman filter1/3(Y_error) -> Transpose3/1, MatrixMultiply1/2, Scope2/1
  B/1 -> kalman filter1/2(B)
  Prelookup/2 -> A/2, steadyState/2, K2/2, K1/2, M/2, L/2, steadyinput/2, steadyOutput/2, D/2, C/2, B/2
  Selector/1 -> Prelookup/1
  steadyState/1 -> kalman filter1/9(Xtrim)
  Transpose3/1 -> Matrix Divide1/1
  Matrix Divide1/1 -> MatrixMultiply1/1
  L/1 -> kalman filter1/10(L)
  C/1 -> kalman filter1/3(C)
  Minus5/1 -> kalman filter1/7(Y)
  kalman filter1/2(Y_es) -> Out1/1
  Minus1/1 -> kalman filter1/8(U)
  kalman filter1/1(X_es) -> Selector/1
  steadyinput/1 -> Minus1/2
  K1/1 -> kalman filter1/5(K)
  steadyOutput/1 -> Minus5/2
  A/1 -> kalman filter1/1(A)
  MatrixMultiply1/1 -> Out2/1
  M/1 -> kalman filter1/11(M)
  In3/1 -> kalman filter1/6(x0)
  In2/1 -> Minus5/1
  In1/1 -> Minus1/1
  K2/1 -> Matrix Divide1/2

== system sensor_diagnosis/NO7 ==
  In1 : Inport
  In2 : Inport  Port=2
  In3 : Inport  Port=3
  In4 : Inport  Port=4
  A : sharedschedule/Interpolate Matrix(x)   matrix=piece.A  aMode=aMode
      settings: SourceProductName=Aerospace Blockset  SourceProductBaseCode=AE
  B : sharedschedule/Interpolate Matrix(x)   matrix=piece.B  aMode=aMode
      settings: SourceProductName=Aerospace Blockset  SourceProductBaseCode=AE
  C : sharedschedule/Interpolate Matrix(x)   matrix=piece.C  aMode=aMode
      settings: SourceProductName=Aerospace Blockset  SourceProductBaseCode=AE
  Constant7 : Constant  Value=R  VectorParams1D=off
  D : sharedschedule/Interpolate Matrix(x)   matrix=piece.D  aMode=aMode
      settings: SourceProductName=Aerospace Blockset  SourceProductBaseCode=AE
  K1 : sharedschedule/Interpolate Matrix(x)   matrix=piece.K_s  aMode=aMode
      settings: SourceProductName=Aerospace Blockset  SourceProductBaseCode=AE
  K2 : sharedschedule/Interpolate Matrix(x)   matrix=piece.S_s  aMode=aMode
      settings: SourceProductName=Aerospace Blockset  SourceProductBaseCode=AE
  L : sharedschedule/Interpolate Matrix(x)   matrix=piece.L  aMode=aMode
      settings: SourceProductName=Aerospace Blockset  SourceProductBaseCode=AE
  M : sharedschedule/Interpolate Matrix(x)   matrix=piece.M  aMode=aMode
      settings: SourceProductName=Aerospace Blockset  SourceProductBaseCode=AE
  Matrix Divide1 : Product  Inputs=*/  Multiplication=Matrix(*)
  MatrixMultiply1 : Product  Multiplication=Matrix(*)
  Minus1 : Sum  Inputs=+-
  Minus5 : Sum  Inputs=+-
  Prelookup : PreLookup  BreakpointsData=piece.Nl  BreakpointObject=Nl  ExtrapMethod=Linear  UseLastBreakpoint=on  DiagnosticForOutOfRangeInput=Warning
  Scope2 : Scope
  Selector : Selector  InputPortWidth=2  IndexOptions=Index vector (dialog)  Indices=[1]  OutputSizes=1
  Transpose3 : Math  Operator=transpose  SaturateOnIntegerOverflow=on
  kalman filter1 : Subsystem
  steadyOutput : sharedschedule/Interpolate Matrix(x)   matrix=piece.steadyOutput  aMode=aMode
      settings: SourceProductName=Aerospace Blockset  SourceProductBaseCode=AE
  steadyState : sharedschedule/Interpolate Matrix(x)   matrix=piece.steadyState  aMode=aMode
      settings: SourceProductName=Aerospace Blockset  SourceProductBaseCode=AE
  steadyinput : sharedschedule/Interpolate Matrix(x)   matrix=piece.steadyInput  aMode=aMode
      settings: SourceProductName=Aerospace Blockset  SourceProductBaseCode=AE
  Out1 : Outport
  Out2 : Outport  Port=2
  wires:
  D/1 -> kalman filter1/4(D)
  Prelookup/1 -> K2/1, K1/1, M/1, L/1, steadyState/1, steadyinput/1, steadyOutput/1, D/1, C/1, B/1, A/1
  In4/1 -> kalman filter1/12(P)
  kalman filter1/3(Y_error) -> Transpose3/1, MatrixMultiply1/2, Scope2/1
  B/1 -> kalman filter1/2(B)
  Prelookup/2 -> A/2, steadyState/2, K2/2, K1/2, M/2, L/2, steadyinput/2, steadyOutput/2, D/2, C/2, B/2
  Selector/1 -> Prelookup/1
  steadyState/1 -> kalman filter1/9(Xtrim)
  Transpose3/1 -> Matrix Divide1/1
  Matrix Divide1/1 -> MatrixMultiply1/1
  L/1 -> kalman filter1/10(L)
  C/1 -> kalman filter1/3(C)
  Minus5/1 -> kalman filter1/7(Y)
  kalman filter1/2(Y_es) -> Out1/1
  Minus1/1 -> kalman filter1/8(U)
  kalman filter1/1(X_es) -> Selector/1
  steadyinput/1 -> Minus1/2
  K1/1 -> kalman filter1/5(K)
  steadyOutput/1 -> Minus5/2
  A/1 -> kalman filter1/1(A)
  MatrixMultiply1/1 -> Out2/1
  M/1 -> kalman filter1/11(M)
  In3/1 -> kalman filter1/6(x0)
  In2/1 -> Minus5/1
  In1/1 -> Minus1/1
  K2/1 -> Matrix Divide1/2

== system sensor_diagnosis/NO8 ==
  In1 : Inport
  In2 : Inport  Port=2
  In3 : Inport  Port=3
  In4 : Inport  Port=4
  A : sharedschedule/Interpolate Matrix(x)   matrix=piece.A  aMode=aMode
      settings: SourceProductName=Aerospace Blockset  SourceProductBaseCode=AE
  B : sharedschedule/Interpolate Matrix(x)   matrix=piece.B  aMode=aMode
      settings: SourceProductName=Aerospace Blockset  SourceProductBaseCode=AE
  C : sharedschedule/Interpolate Matrix(x)   matrix=piece.C  aMode=aMode
      settings: SourceProductName=Aerospace Blockset  SourceProductBaseCode=AE
  Constant7 : Constant  Value=R  VectorParams1D=off
  D : sharedschedule/Interpolate Matrix(x)   matrix=piece.D  aMode=aMode
      settings: SourceProductName=Aerospace Blockset  SourceProductBaseCode=AE
  K1 : sharedschedule/Interpolate Matrix(x)   matrix=piece.K_s  aMode=aMode
      settings: SourceProductName=Aerospace Blockset  SourceProductBaseCode=AE
  K2 : sharedschedule/Interpolate Matrix(x)   matrix=piece.S_s  aMode=aMode
      settings: SourceProductName=Aerospace Blockset  SourceProductBaseCode=AE
  L : sharedschedule/Interpolate Matrix(x)   matrix=piece.L  aMode=aMode
      settings: SourceProductName=Aerospace Blockset  SourceProductBaseCode=AE
  M : sharedschedule/Interpolate Matrix(x)   matrix=piece.M  aMode=aMode
      settings: SourceProductName=Aerospace Blockset  SourceProductBaseCode=AE
  Matrix Divide1 : Product  Inputs=*/  Multiplication=Matrix(*)
  MatrixMultiply1 : Product  Multiplication=Matrix(*)
  Minus1 : Sum  Inputs=+-
  Minus5 : Sum  Inputs=+-
  Prelookup : PreLookup  BreakpointsData=piece.Nl  BreakpointObject=Nl  ExtrapMethod=Linear  UseLastBreakpoint=on  DiagnosticForOutOfRangeInput=Warning
  Scope2 : Scope
  Selector : Selector  InputPortWidth=2  IndexOptions=Index vector (dialog)  Indices=[1]  OutputSizes=1
  Transpose3 : Math  Operator=transpose  SaturateOnIntegerOverflow=on
  kalman filter1 : Subsystem
  steadyOutput : sharedschedule/Interpolate Matrix(x)   matrix=piece.steadyOutput  aMode=aMode
      settings: SourceProductName=Aerospace Blockset  SourceProductBaseCode=AE
  steadyState : sharedschedule/Interpolate Matrix(x)   matrix=piece.steadyState  aMode=aMode
      settings: SourceProductName=Aerospace Blockset  SourceProductBaseCode=AE
  steadyinput : sharedschedule/Interpolate Matrix(x)   matrix=piece.steadyInput  aMode=aMode
      settings: SourceProductName=Aerospace Blockset  SourceProductBaseCode=AE
  Out1 : Outport
  Out2 : Outport  Port=2
  wires:
  D/1 -> kalman filter1/4(D)
  Prelookup/1 -> K2/1, K1/1, M/1, L/1, steadyState/1, steadyinput/1, steadyOutput/1, D/1, C/1, B/1, A/1
  In4/1 -> kalman filter1/12(P)
  kalman filter1/3(Y_error) -> Transpose3/1, MatrixMultiply1/2, Scope2/1
  B/1 -> kalman filter1/2(B)
  Prelookup/2 -> A/2, steadyState/2, K2/2, K1/2, M/2, L/2, steadyinput/2, steadyOutput/2, D/2, C/2, B/2
  Selector/1 -> Prelookup/1
  steadyState/1 -> kalman filter1/9(Xtrim)
  Transpose3/1 -> Matrix Divide1/1
  Matrix Divide1/1 -> MatrixMultiply1/1
  L/1 -> kalman filter1/10(L)
  C/1 -> kalman filter1/3(C)
  Minus5/1 -> kalman filter1/7(Y)
  kalman filter1/2(Y_es) -> Out1/1
  Minus1/1 -> kalman filter1/8(U)
  kalman filter1/1(X_es) -> Selector/1
  steadyinput/1 -> Minus1/2
  K1/1 -> kalman filter1/5(K)
  steadyOutput/1 -> Minus5/2
  A/1 -> kalman filter1/1(A)
  MatrixMultiply1/1 -> Out2/1
  M/1 -> kalman filter1/11(M)
  In3/1 -> kalman filter1/6(x0)
  In2/1 -> Minus5/1
  In1/1 -> Minus1/1
  K2/1 -> Matrix Divide1/2

== system sensor_diagnosis/NO9 ==
  In1 : Inport
  In2 : Inport  Port=2
  In3 : Inport  Port=3
  In4 : Inport  Port=4
  A : sharedschedule/Interpolate Matrix(x)   matrix=piece.A  aMode=aMode
      settings: SourceProductName=Aerospace Blockset  SourceProductBaseCode=AE
  B : sharedschedule/Interpolate Matrix(x)   matrix=piece.B  aMode=aMode
      settings: SourceProductName=Aerospace Blockset  SourceProductBaseCode=AE
  C : sharedschedule/Interpolate Matrix(x)   matrix=piece.C  aMode=aMode
      settings: SourceProductName=Aerospace Blockset  SourceProductBaseCode=AE
  Constant7 : Constant  Value=R  VectorParams1D=off
  D : sharedschedule/Interpolate Matrix(x)   matrix=piece.D  aMode=aMode
      settings: SourceProductName=Aerospace Blockset  SourceProductBaseCode=AE
  K1 : sharedschedule/Interpolate Matrix(x)   matrix=piece.K_s  aMode=aMode
      settings: SourceProductName=Aerospace Blockset  SourceProductBaseCode=AE
  K2 : sharedschedule/Interpolate Matrix(x)   matrix=piece.S_s  aMode=aMode
      settings: SourceProductName=Aerospace Blockset  SourceProductBaseCode=AE
  L : sharedschedule/Interpolate Matrix(x)   matrix=piece.L  aMode=aMode
      settings: SourceProductName=Aerospace Blockset  SourceProductBaseCode=AE
  M : sharedschedule/Interpolate Matrix(x)   matrix=piece.M  aMode=aMode
      settings: SourceProductName=Aerospace Blockset  SourceProductBaseCode=AE
  Matrix Divide1 : Product  Inputs=*/  Multiplication=Matrix(*)
  MatrixMultiply1 : Product  Multiplication=Matrix(*)
  Minus1 : Sum  Inputs=+-
  Minus5 : Sum  Inputs=+-
  Prelookup : PreLookup  BreakpointsData=piece.Nl  BreakpointObject=Nl  ExtrapMethod=Linear  UseLastBreakpoint=on  DiagnosticForOutOfRangeInput=Warning
  Scope2 : Scope
  Selector : Selector  InputPortWidth=2  IndexOptions=Index vector (dialog)  Indices=[1]  OutputSizes=1
  Transpose3 : Math  Operator=transpose  SaturateOnIntegerOverflow=on
  kalman filter1 : Subsystem
  steadyOutput : sharedschedule/Interpolate Matrix(x)   matrix=piece.steadyOutput  aMode=aMode
      settings: SourceProductName=Aerospace Blockset  SourceProductBaseCode=AE
  steadyState : sharedschedule/Interpolate Matrix(x)   matrix=piece.steadyState  aMode=aMode
      settings: SourceProductName=Aerospace Blockset  SourceProductBaseCode=AE
  steadyinput : sharedschedule/Interpolate Matrix(x)   matrix=piece.steadyInput  aMode=aMode
      settings: SourceProductName=Aerospace Blockset  SourceProductBaseCode=AE
  Out1 : Outport
  Out2 : Outport  Port=2
  wires:
  D/1 -> kalman filter1/4(D)
  Prelookup/1 -> K2/1, K1/1, M/1, L/1, steadyState/1, steadyinput/1, steadyOutput/1, D/1, C/1, B/1, A/1
  In4/1 -> kalman filter1/12(P)
  kalman filter1/3(Y_error) -> Transpose3/1, MatrixMultiply1/2, Scope2/1
  B/1 -> kalman filter1/2(B)
  Prelookup/2 -> A/2, steadyState/2, K2/2, K1/2, M/2, L/2, steadyinput/2, steadyOutput/2, D/2, C/2, B/2
  Selector/1 -> Prelookup/1
  steadyState/1 -> kalman filter1/9(Xtrim)
  Transpose3/1 -> Matrix Divide1/1
  Matrix Divide1/1 -> MatrixMultiply1/1
  L/1 -> kalman filter1/10(L)
  C/1 -> kalman filter1/3(C)
  Minus5/1 -> kalman filter1/7(Y)
  kalman filter1/2(Y_es) -> Out1/1
  Minus1/1 -> kalman filter1/8(U)
  kalman filter1/1(X_es) -> Selector/1
  steadyinput/1 -> Minus1/2
  K1/1 -> kalman filter1/5(K)
  steadyOutput/1 -> Minus5/2
  A/1 -> kalman filter1/1(A)
  MatrixMultiply1/1 -> Out2/1
  M/1 -> kalman filter1/11(M)
  In3/1 -> kalman filter1/6(x0)
  In2/1 -> Minus5/1
  In1/1 -> Minus1/1
  K2/1 -> Matrix Divide1/2

== system sensor_diagnosis/Subsystem2 ==
  signal : Inport
  Band-Limited White Noise : simulink/Sources/Band-Limited White Noise  Cov=ones(3,1)*0.0025^2*0.02  Ts=0.02  seed=[1000:500:2000]
  Constant7 : Constant  Value=0.002
  Multiply : Product
  Sum7 : Sum  Inputs=|++
  signal with noise : Outport
  wires:
  Band-Limited White Noise/1 -> Multiply/1
  Sum7/1 -> signal with noise/1
  signal/1 -> Sum7/1
  Multiply/1 -> Sum7/2
  Constant7/1 -> Multiply/2

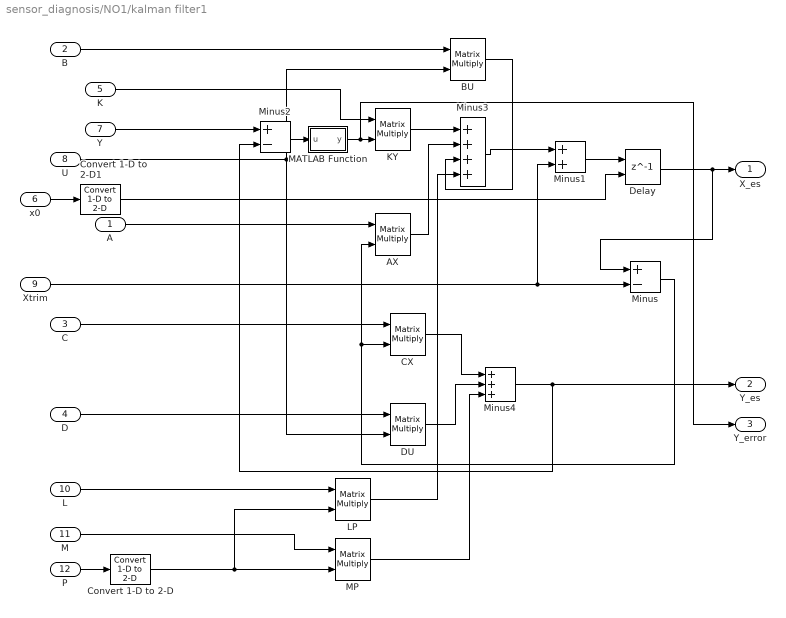
== system sensor_diagnosis/NO1/kalman filter1 ==
  A : Inport
  B : Inport  Port=2
  C : Inport  Port=3
  D : Inport  Port=4
  K : Inport  Port=5
  x0 : Inport  Port=6
  Y : Inport  Port=7
  U : Inport  Port=8
  Xtrim : Inport  Port=9
  L : Inport  Port=10
  M : Inport  Port=11
  P : Inport  Port=12
  "\tCX" : Product  Multiplication=Matrix(*)
  AX : Product  Multiplication=Matrix(*)
  BU : Product  Multiplication=Matrix(*)
  Convert 1-D to 2-D : dspsigattribs/Convert 1-D to 2-D  M=10  N=1  frameBasedOut=off
      settings: SourceProductName=DSP System Toolbox  SourceProductBaseCode=DS
  Convert 1-D to 2-D1 : dspsigattribs/Convert 1-D to 2-D  M=2  N=1  frameBasedOut=off
      settings: SourceProductName=DSP System Toolbox  SourceProductBaseCode=DS
  DU : Product  Multiplication=Matrix(*)
  Delay : Delay  DelayLength=1  InitialConditionSource=Input port
      settings: InputPortMap=u0,p4
  KY : Product  Multiplication=Matrix(*)
  LP : Product  Multiplication=Matrix(*)
  MATLAB Function : MATLAB Function  TreatAsAtomicUnit=on
  MP : Product  Multiplication=Matrix(*)
  Minus : Sum  Inputs=+-
  Minus1 : Sum
  Minus2 : Sum  Inputs=+-
  Minus3 : Sum  Inputs=++++
  Minus4 : Sum  Inputs=+++
  X_es : Outport
  Y_es : Outport  Port=2
  Y_error : Outport  Port=3
  wires:
  Minus1/1 -> Delay/1
  Minus3/1 -> Minus1/1
  AX/1 -> Minus3/2
  Minus/1 -> "\tCX"/2, AX/2
  Delay/1 -> X_es/1, Minus/1
  Xtrim/1 -> Minus/2, Minus1/2
  K/1 -> KY/1
  D/1 -> DU/1
  C/1 -> "\tCX"/1
  B/1 -> BU/1
  A/1 -> AX/1
  BU/1 -> Minus3/3
  "\tCX"/1 -> Minus4/1
  DU/1 -> Minus4/2
  Y/1 -> Minus2/1
  U/1 -> DU/2, BU/2
  KY/1 -> Minus3/1
  Minus4/1 -> Y_es/1, Minus2/2
  L/1 -> LP/1
  M/1 -> MP/1
  LP/1 -> Minus3/4
  MP/1 -> Minus4/3
  P/1 -> Convert 1-D to 2-D/1
  Convert 1-D to 2-D/1 -> LP/2, MP/2
  x0/1 -> Convert 1-D to 2-D1/1
  Convert 1-D to 2-D1/1 -> Delay/2
  Minus2/1 -> MATLAB Function/1(u)
  MATLAB Function/1(y) -> Y_error/1, KY/2
